simulink model "PIDPWMHopper"  (R2023b)
settings: Solver=VariableStepAuto  StartTime=0.0  StopTime=10  RelTol=1e-3
values from neighbouring files (symbols this model uses):
  controlInput = 10.2    [PIDPWM_HopperSim_Take2.m]
  desiredVel = 0    [PIDPWM_HopperSim_Take2.m]
  finalPos = .41    (= 0.41)    [PIDPWM_HopperSim_Take2.m]
  g = -9.81    [PIDPWM_HopperSim_Take2.m]
  initialPos = 0    [PIDPWM_HopperSim_Take2.m]
  kd = 0    [PIDPWM_HopperSim_Take2.m]
  ki = 0    [PIDPWM_HopperSim_Take2.m]
  kp = 30    [PIDPWM_HopperSim_Take2.m]
  m = .091    (= 0.091)    [PIDPWM_HopperSim_Take2.m]
  noiseGain = 0    [PIDPWM_HopperSim_Take2.m]
undefined symbols (not defined in the file or in its folder): finalVal, initialVal, P_pulse, PWM_Visualize_Gain, timeStep
libraries: simulink x1, vrlib x1
settings Model: Creator=benjackson  LastModifiedBy=ben
settings OptimizationCC: ReuseModelBlockBuffer=off

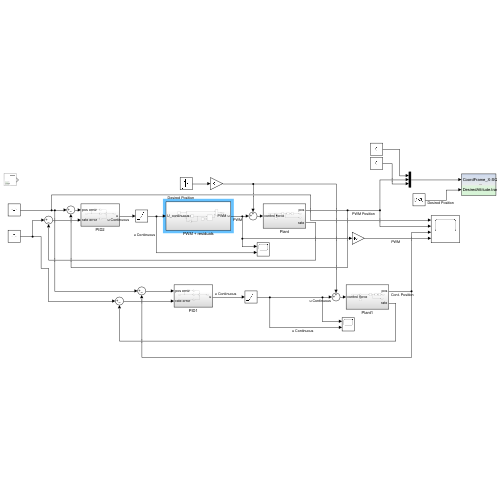
[thumbnail: Simulink's stored preview of the top-level diagram]
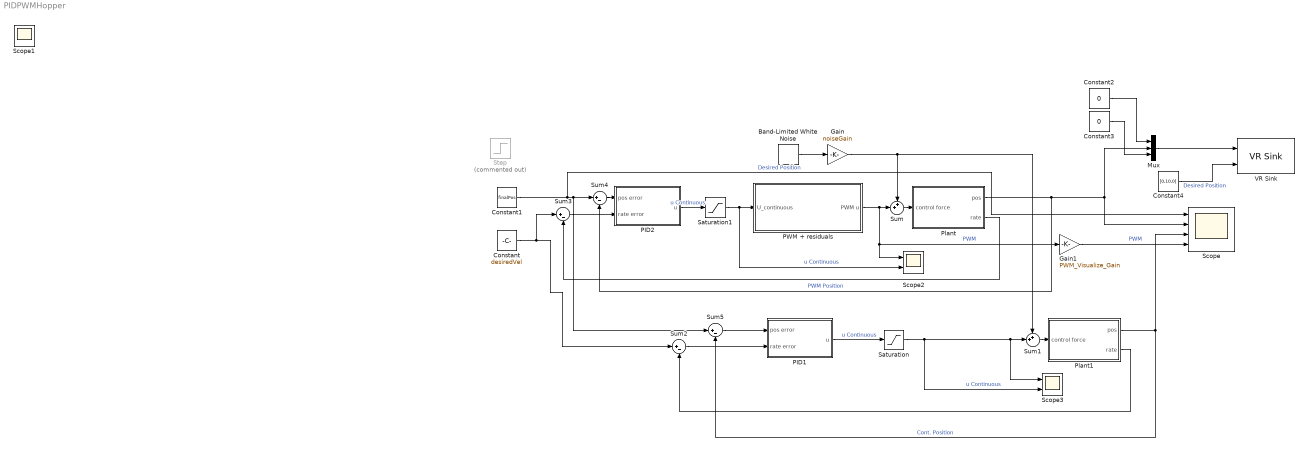
== system PIDPWMHopper ==
  Band-Limited White Noise : simulink/Sources/Band-Limited White Noise  Cov=[0.1]  Ts=1e-3  seed=[23341]
  Constant : Constant  Value=desiredVel
  Constant1 : Constant  Value=finalPos
  Constant2 : Constant  Value=0
  Constant3 : Constant  Value=0
  Constant4 : Constant  Value=[0,10,0]
  Gain : Gain  Gain=noiseGain
  Gain1 : Gain  Gain=PWM_Visualize_Gain
  Mux : Mux  Inputs=3
  PID1 : Subsystem
  PID2 : Subsystem
  PWM + residuals : Subsystem
  Plant : Subsystem
  Plant1 : Subsystem
  Saturation : Saturate  UpperLimit=1000  LowerLimit=0
  Saturation1 : Saturate  UpperLimit=1000  LowerLimit=0
  Scope : Scope  NumInputPorts=4
  Scope2 : Scope  NumInputPorts=2
  Scope3 : Scope  NumInputPorts=2
  Step : Step  Commented=on  Time=timeStep  Before=initialVal  After=finalVal  SampleTime=0
  Sum : Sum  Inputs=++|
  Sum1 : Sum  Inputs=++|
  Sum{2..5} (4 alike) : Sum  Inputs=|+-
  VR Sink : vrlib/VR Sink  InstantiateOnLoad=on  SampleTime=0.1  ViewEnable=on  RemoteChange=off  RemoteView=off  FieldsWritten=CoordFrame_X-SQUARE_Y-CIRCLE_Z-OCTOGO_Transform.translation.3.1.1.double#DesiredAttitude.translation.3.1.1.double  WorldFileName=World.x3d  WorldDescription=Straight Road Strip - 2 Lanes  AutoView=off  VideoDimensions=[]  AllowVariableSize=off
  Scope1 : Scope
  wires:
  Sum4/1 -> PID2/1(pos error)
  Sum3/1 -> PID2/2(rate error)
  Plant/2(rate) -> Sum3/2
  Band-Limited White Noise/1 -> Gain/1
  Plant/1(pos) -> Scope/2, Mux/2, Sum4/2  "PWM Position"
  Sum/1 -> Plant/1(control force)
  PWM + residuals/1(PWM u) -> Scope2/1, Gain1/1, Sum/2  "PWM"
  Sum5/1 -> PID1/1(pos error)
  Plant1/2(rate) -> Sum2/2
  Plant1/1(pos) -> Sum5/2, Scope/3  "Cont. Position"
  Saturation/1 -> Scope3/2, Scope3/1, Sum1/2  "u Continuous"
  Constant1/1 -> Sum5/1, Sum4/1, Scope/1  "Desired Position"
  Sum2/1 -> PID1/2(rate error)
  Sum1/1 -> Plant1/1(control force)
  Gain/1 -> Sum/1, Sum1/1
  Constant/1 -> Sum2/1, Sum3/1
  Gain1/1 -> Scope/4  "PWM"
  PID1/1(u) -> Saturation/1  "u Continuous"
  PID2/1(u) -> Saturation1/1  "u Continuous"
  Saturation1/1 -> Scope2/2, PWM + residuals/1(U_continuous)  "u Continuous"
  Constant3/1 -> Mux/3
  Constant2/1 -> Mux/1
  Mux/1 -> VR Sink/1
  Constant4/1 -> VR Sink/2  "Desired Position"

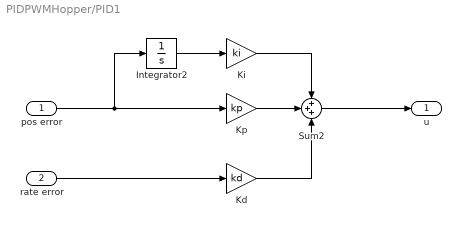
== system PIDPWMHopper/PID1 ==
  pos error : Inport
  rate error : Inport  Port=2
  Integrator2 : Integrator
  Kd : Gain  Gain=kd
  Ki : Gain  Gain=ki
  Kp : Gain  Gain=kp
  Sum2 : Sum  Inputs=+++
  u : Outport
  wires:
  Sum2/1 -> u/1
  rate error/1 -> Kd/1
  Ki/1 -> Sum2/1
  pos error/1 -> Integrator2/1, Kp/1
  Integrator2/1 -> Ki/1
  Kd/1 -> Sum2/3
  Kp/1 -> Sum2/2

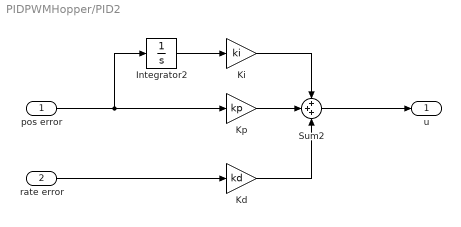
== system PIDPWMHopper/PID2 ==
  pos error : Inport
  rate error : Inport  Port=2
  Integrator2 : Integrator
  Kd : Gain  Gain=kd
  Ki : Gain  Gain=ki
  Kp : Gain  Gain=kp
  Sum2 : Sum  Inputs=+++
  u : Outport
  wires:
  Sum2/1 -> u/1
  rate error/1 -> Kd/1
  Ki/1 -> Sum2/1
  pos error/1 -> Integrator2/1, Kp/1
  Integrator2/1 -> Ki/1
  Kd/1 -> Sum2/3
  Kp/1 -> Sum2/2

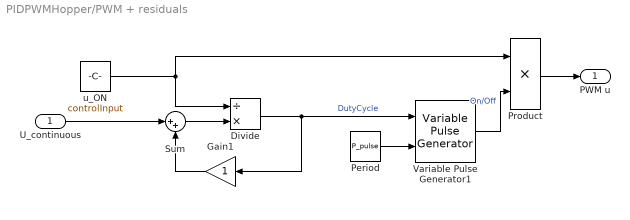
== system PIDPWMHopper/PWM + residuals ==
  U_continuous : Inport
  Divide : Product  Inputs=/*
  Gain1 : Gain
  Period : Constant  Value=P_pulse
  Product : Product
  Sum : Sum  Inputs=|++
  Variable Pulse Generator1 : VariablePulseGenerator  AllowZeroPulseWidth=on  SampleTime=0.1
  u_ON : Constant  Value=controlInput
  PWM u : Outport
  wires:
  U_continuous/1 -> Sum/1
  Divide/1 -> Gain1/1, Variable Pulse Generator1/1  "DutyCycle"
  Gain1/1 -> Sum/2
  Sum/1 -> Divide/2
  Product/1 -> PWM u/1
  u_ON/1 -> Product/1, Divide/1
  Variable Pulse Generator1/1 -> Product/2  "On/Off"
  Period/1 -> Variable Pulse Generator1/2

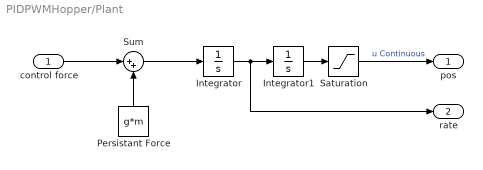
== system PIDPWMHopper/Plant ==
  control force : Inport
  Integrator : Integrator
  Integrator1 : Integrator  InitialCondition=initialPos
  Persistant Force : Constant  Value=g*m
  Saturation : Saturate  UpperLimit=1000  LowerLimit=0
  Sum : Sum  Inputs=|++
  pos : Outport
  rate : Outport  Port=2
  wires:
  control force/1 -> Sum/1
  Integrator/1 -> rate/1, Integrator1/1
  Sum/1 -> Integrator/1
  Persistant Force/1 -> Sum/2
  Integrator1/1 -> Saturation/1
  Saturation/1 -> pos/1  "u Continuous"

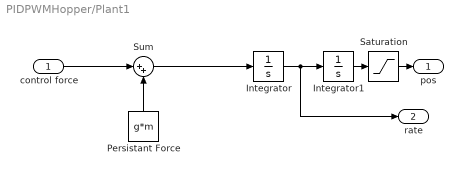
== system PIDPWMHopper/Plant1 ==
  control force : Inport
  Integrator : Integrator
  Integrator1 : Integrator  InitialCondition=initialPos
  Persistant Force : Constant  Value=g*m
  Saturation : Saturate  UpperLimit=1000  LowerLimit=0
  Sum : Sum  Inputs=|++
  pos : Outport
  rate : Outport  Port=2
  wires:
  control force/1 -> Sum/1
  Integrator1/1 -> Saturation/1
  Integrator/1 -> rate/1, Integrator1/1
  Sum/1 -> Integrator/1
  Persistant Force/1 -> Sum/2
  Saturation/1 -> pos/1
